simulink model "Y_FK_mdl"  (R2013a)
settings: Solver=ode45  StartTime=0.0  StopTime=inf  RelTol=1e-3
undefined symbols (not defined in the file or in its folder): ToSimulink_Y_FK_ST, ToSimulink_Y_Signals2VRML
libraries: simulink x5, vrlib x1
settings Model: Creator=Jose Angel Rangel  LastModifiedBy=Jose Angel Rangel

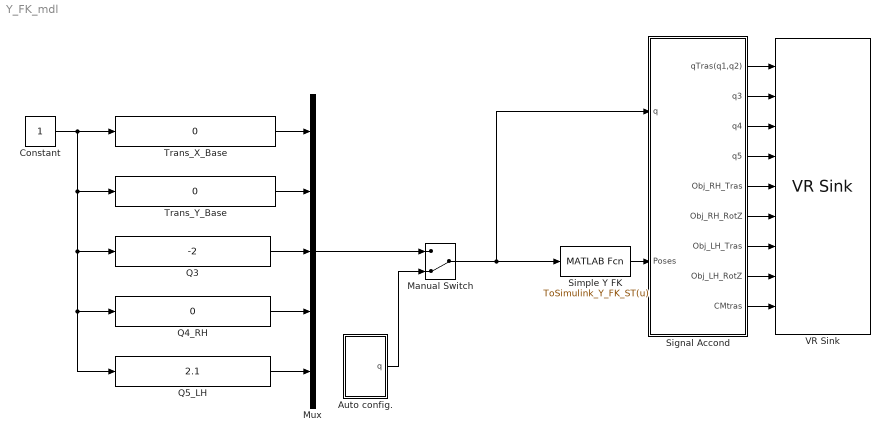
== system Y_FK_mdl ==
  Auto config. : Subsystem
  Constant : Constant
  Manual Switch : ManualSwitch  CurrentSetting=0
  Mux : Mux  Inputs=5
  Q3 : simulink/Math Operations/Slider Gain  low=-5  gain=-2  high=5
  Q4_RH : simulink/Math Operations/Slider Gain  low=-5  gain=0  high=5
  Q5_LH : simulink/Math Operations/Slider Gain  low=-5  gain=2.1  high=5
  Signal Accond : Subsystem
  Simple Y FK : MATLABFcn  MATLABFcn=ToSimulink_Y_FK_ST(u)
  Trans_X_Base : simulink/Math Operations/Slider Gain  low=-5  gain=0  high=5
  Trans_Y_Base : simulink/Math Operations/Slider Gain  low=-5  gain=0  high=5
  VR Sink : vrlib/VR Sink  InstantiateOnLoad=on  SampleTime=0.1  ViewEnable=on  RemoteChange=off  RemoteView=off  FieldsWritten=Base_Tras.translation.3.1.1.double#Base_Rot.rotation.4.1.1.double#Q4.rotation.4.1.1.double#Q5.rotation.4.1.1.double#Obj_RH.translation.3.1.1.double#Rot_Obj_RH.rotation.4.1.1.double#Obj_LH.translation.3.1.1.double#Rot_Obj_LH.rotation.4.1.1.double#Actual_CM.translation.3.1.1.double  WorldFileName=Simpley.wrl  AutoView=on  VideoDimensions=[]  AllowVariableSize=off
  wires:
  Constant/1 -> Q5_LH/1, Q4_RH/1, Q3/1, Trans_Y_Base/1, Trans_X_Base/1
  Q5_LH/1 -> Mux/5
  Q4_RH/1 -> Mux/4
  Q3/1 -> Mux/3
  Trans_Y_Base/1 -> Mux/2
  Trans_X_Base/1 -> Mux/1
  Mux/1 -> Manual Switch/1
  Auto config./1(q) -> Manual Switch/2
  Manual Switch/1 -> Simple Y FK/1, Signal Accond/1(q)
  Simple Y FK/1 -> Signal Accond/2(Poses)
  Signal Accond/8(Obj_LH_RotZ) -> VR Sink/8
  Signal Accond/7("Obj_LH_Tras ") -> VR Sink/7
  Signal Accond/9(CMtras) -> VR Sink/9
  Signal Accond/5(Obj_RH_Tras) -> VR Sink/5
  Signal Accond/2(q3) -> VR Sink/2
  Signal Accond/3(q4) -> VR Sink/3
  Signal Accond/1(qTras(q1,q2)) -> VR Sink/1
  Signal Accond/6(Obj_RH_RotZ) -> VR Sink/6
  Signal Accond/4(q5) -> VR Sink/4

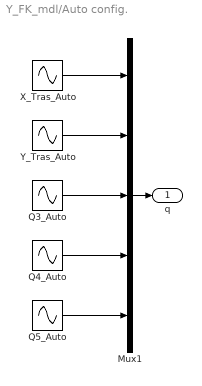
== system Y_FK_mdl/Auto config. ==
  Mux1 : Mux  Inputs=5
  Q3_Auto : Sin  Amplitude=2*pi  Frequency=.5  SampleTime=0
  Q4_Auto : Sin  Amplitude=2*pi  Frequency=.2  SampleTime=0
  Q5_Auto : Sin  Amplitude=2*pi  Frequency=.8  SampleTime=0
  X_Tras_Auto : Sin  Amplitude=2*pi  SampleTime=0
  Y_Tras_Auto : Sin  Amplitude=2*pi  Frequency=1.5  SampleTime=0
  q : Outport
  wires:
  Mux1/1 -> q/1
  X_Tras_Auto/1 -> Mux1/1
  Q3_Auto/1 -> Mux1/3
  Y_Tras_Auto/1 -> Mux1/2
  Q4_Auto/1 -> Mux1/4
  Q5_Auto/1 -> Mux1/5

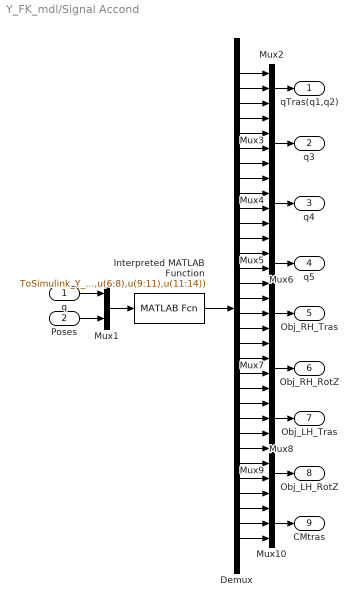
== system Y_FK_mdl/Signal Accond ==
  q : Inport
  Poses : Inport  Port=2
  Demux : Demux  Outputs=32
  Interpreted MATLAB Function : MATLABFcn  MATLABFcn=ToSimulink_Y_Signals2VRML(u(1:5),u(6:8),u(9:11),u(11:14))
  Mux1 : Mux  Inputs=2
  Mux{2,6,8,10} (4 alike) : Mux  Inputs=3
  Mux{3..5,7,9} (5 alike) : Mux
  qTras(q1,q2) : Outport
  q3 : Outport  Port=2
  q4 : Outport  Port=3
  q5 : Outport  Port=4
  Obj_RH_Tras : Outport  Port=5
  Obj_RH_RotZ : Outport  Port=6
  "Obj_LH_Tras " : Outport  Port=7
  Obj_LH_RotZ : Outport  Port=8
  CMtras : Outport  Port=9
  wires:
  Mux6/1 -> Obj_RH_Tras/1
  Mux4/1 -> q4/1
  Mux1/1 -> Interpreted MATLAB Function/1
  Mux5/1 -> q5/1
  Mux10/1 -> CMtras/1
  Mux2/1 -> qTras(q1,q2)/1
  Mux9/1 -> Obj_LH_RotZ/1
  Mux8/1 -> "Obj_LH_Tras "/1
  Mux3/1 -> q3/1
  Mux7/1 -> Obj_RH_RotZ/1
  Demux/30 -> Mux10/1
  Demux/7 -> Mux3/4
  Demux/3 -> Mux2/3
  Demux/16 -> Mux6/1
  Demux/13 -> Mux5/2
  Demux/31 -> Mux10/2
  Demux/5 -> Mux3/2
  Demux/14 -> Mux5/3
  Demux/17 -> Mux6/2
  Demux/20 -> Mux7/2
  Demux/11 -> Mux4/4
  Demux/4 -> Mux3/1
  Demux/27 -> Mux9/2
  Demux/8 -> Mux4/1
  Demux/15 -> Mux5/4
  Demux/26 -> Mux9/1
  Demux/18 -> Mux6/3
  Demux/10 -> Mux4/3
  Demux/24 -> Mux8/2
  Demux/9 -> Mux4/2
  Demux/6 -> Mux3/3
  Demux/28 -> Mux9/3
  Demux/32 -> Mux10/3
  Interpreted MATLAB Function/1 -> Demux/1
  Demux/25 -> Mux8/3
  Poses/1 -> Mux1/2
  Demux/12 -> Mux5/1
  Demux/23 -> Mux8/1
  Demux/22 -> Mux7/4
  Demux/19 -> Mux7/1
  Demux/21 -> Mux7/3
  Demux/29 -> Mux9/4
  Demux/2 -> Mux2/2
  Demux/1 -> Mux2/1
  q/1 -> Mux1/1
